simulink model "FonctionBFenZ_et_correcteur_isole"  (R2020a)
settings: Solver=VariableStepAuto  StartTime=0.0  StopTime=0.04  RelTol=1e-3
values from neighbouring files (symbols this model uses):
  denCD = [Rmoteur*tm Rmoteur]    [correcteur.m]
  denCR = [t1*t2 t1+t2 1]    [correcteur.m]
  numCD = [2*E]    [correcteur.m]
  numCR = [Kretour]    [correcteur.m]
  Te = 1/Fe    (= 0.000277777777778)    [correcteur.m]    (also in correcteur2.m)
libraries: cstblocks x2
settings Model: Creator=predon  LastModifiedBy=predon

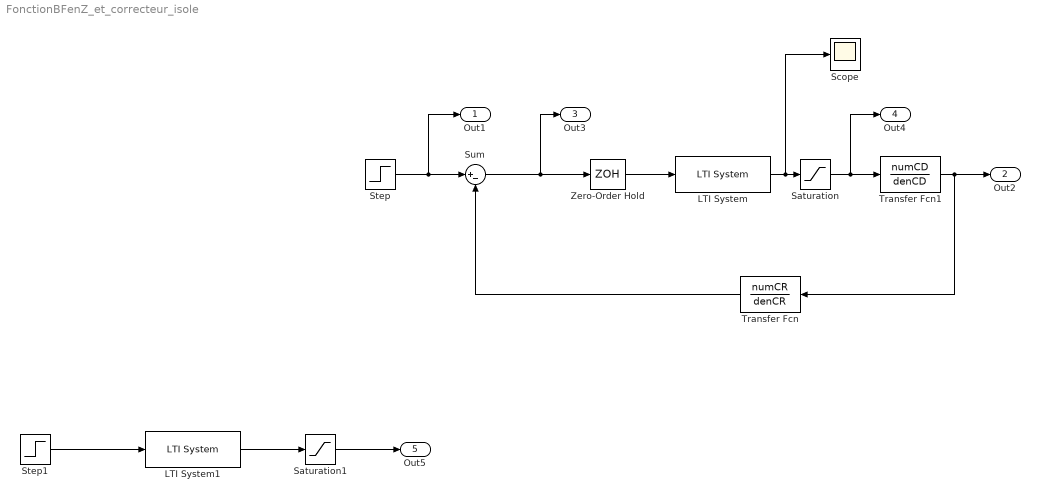
== system FonctionBFenZ_et_correcteur_isole ==
  LTI System : cstblocks/LTI System  sys=Cz  IC=[]
  LTI System1 : cstblocks/LTI System  sys=Cz  IC=[]
  Saturation : Saturate
  Saturation1 : Saturate
  Scope : Scope
  Step : Step  Time=0.02  After=0.5  SampleTime=0
  Step1 : Step  Time=0.02  After=0.1  SampleTime=0
  Sum : Sum  Inputs=|+-
  Transfer Fcn : TransferFcn  Numerator=numCR  Denominator=denCR
  Transfer Fcn1 : TransferFcn  Numerator=numCD  Denominator=denCD
  Zero-Order Hold : ZeroOrderHold  SampleTime=Te
  Out1 : Outport  SignalName=Icons
  Out2 : Outport  Port=2  SignalName=Is
  Out3 : Outport  Port=3  SignalName=Erreur
  Out4 : Outport  Port=4  SignalName=Alpha
  Out5 : Outport  Port=5  SignalName=Is
  wires:
  Transfer Fcn1/1 -> Out2/1, Transfer Fcn/1
  Step/1 -> Out1/1, Sum/1
  Sum/1 -> Zero-Order Hold/1, Out3/1
  Transfer Fcn/1 -> Sum/2
  LTI System/1 -> Scope/1, Saturation/1
  Saturation/1 -> Transfer Fcn1/1, Out4/1
  Zero-Order Hold/1 -> LTI System/1
  Step1/1 -> LTI System1/1
  LTI System1/1 -> Saturation1/1
  Saturation1/1 -> Out5/1
